simulink model "tanks_dis"  (R2021b)
settings: Solver=VariableStepAuto  StartTime=0.0  StopTime=200  RelTol=1e-3
values from neighbouring files (symbols this model uses):
  F = tf([K_pid*(Ti+Td*Ti*N), K_pid*(Ti*N +1),K_pid*N],[Ti, Ti*N 0])    [control_design.m]
  Ts = 4    [control_design.m]
  uss = alpha2/beta*sqrt(2*g*tank_init_h2)*100/15    [control_design.m]
  yss = 40    [control_design.m]
undefined symbols (not defined in the file or in its folder): A_discretized, B_discretized, C_discretized, D_discretized, tank_A1, tank_a1, tank_A2, tank_a2, tank_H1, tank_H2, tank_init_h1, tank_init_h2, tank_Kpump
settings Model: LastModifiedBy=rivaa
settings OptimizationCC: BlockReduction=off  BooleanDataType=off
settings DebuggingCC: SaveWithParameterizedLinksMsg=none  UnderspecifiedInitializationDetection=Classic  MergeDetectMultiDrivingBlocksExec=none  SignalResolutionControl=TryResolveAllWithWarning
settings HardwareCC: TargetUnknown=on
settings ModelReferenceCC: PropagateSignalLabelsOutOfModel=off

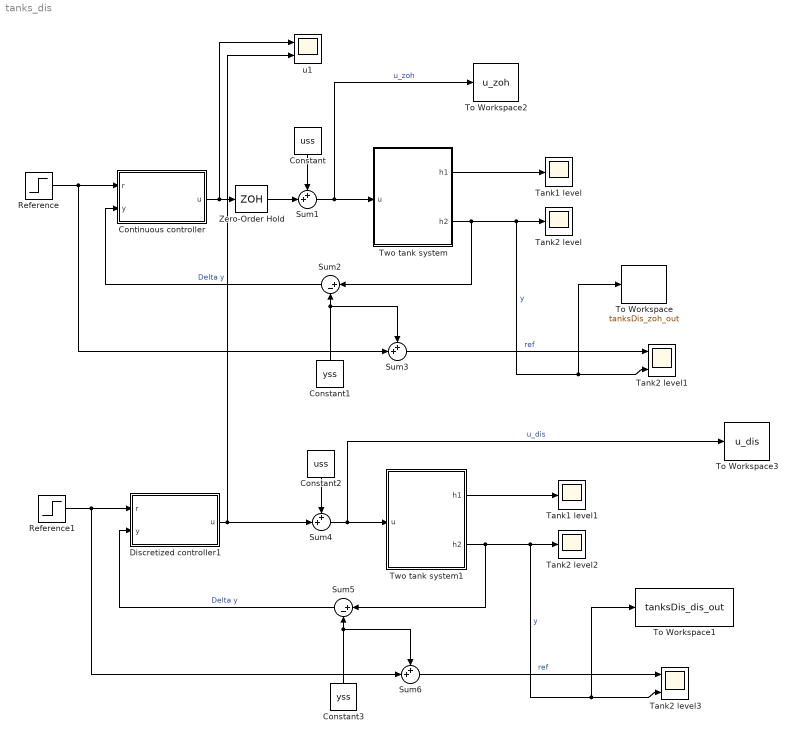
== system tanks_dis ==
  Constant : Constant  Value=uss
  Constant1 : Constant  Value=yss
  Constant2 : Constant  Value=uss
  Constant3 : Constant  Value=yss
  Continuous controller : Subsystem
  Discretized controller1 : Subsystem
  Reference : Step  Time=25  After=10  SampleTime=0
  Reference1 : Step  Time=25  After=10  SampleTime=0
  Sum{1,3..4,6} (4 alike) : Sum  Inputs=++|
  Sum2 : Sum  Inputs=|+-
  Sum5 : Sum  Inputs=|+-
  Tank1 level : Scope
  Tank1 level1 : Scope
  Tank2 level : Scope
  Tank2 level1 : Scope  NumInputPorts=2
  Tank2 level2 : Scope
  Tank2 level3 : Scope  NumInputPorts=2
  To Workspace : ToWorkspace  VariableName=tanksDis_zoh_out  SaveFormat=Structure With Time  SampleTime=-1
      settings: Save2DSignal=2-D array (concatenate along first dimension)
  To Workspace1 : ToWorkspace  VariableName=tanksDis_dis_out  SaveFormat=Structure With Time  SampleTime=-1
      settings: Save2DSignal=2-D array (concatenate along first dimension)
  To Workspace2 : ToWorkspace  VariableName=u_zoh  SaveFormat=Structure With Time  SampleTime=-1
      settings: Save2DSignal=2-D array (concatenate along first dimension)
  To Workspace3 : ToWorkspace  VariableName=u_dis  SaveFormat=Structure With Time  SampleTime=-1
      settings: Save2DSignal=2-D array (concatenate along first dimension)
  Two tank system : Subsystem
  Two tank system1 : Subsystem
  Zero-Order Hold : ZeroOrderHold  SampleTime=Ts
  u1 : Scope  NumInputPorts=2
  wires:
  Constant1/1 -> Sum3/1, Sum2/2
  Continuous controller/1(u) -> u1/1, Zero-Order Hold/1
  Constant/1 -> Sum1/1
  Two tank system/1(h1) -> Tank1 level/1
  Sum1/1 -> To Workspace2/1, Two tank system/1(u)  "u_zoh"
  Two tank system/2(h2) -> Sum2/1, To Workspace/1, Tank2 level1/2, Tank2 level/1  "y"
  Zero-Order Hold/1 -> Sum1/2
  Reference/1 -> Continuous controller/1(r), Sum3/2
  Sum3/1 -> Tank2 level1/1  "ref"
  Sum2/1 -> Continuous controller/2(y)  "Delta y"
  Sum5/1 -> Discretized controller1/2(y)  "Delta y"
  Sum6/1 -> Tank2 level3/1  "ref"
  Reference1/1 -> Discretized controller1/1(r), Sum6/2
  Discretized controller1/1(u) -> u1/2, Sum4/2
  Two tank system1/2(h2) -> Tank2 level2/1, Tank2 level3/2, To Workspace1/1, Sum5/1  "y"
  Sum4/1 -> To Workspace3/1, Two tank system1/1(u)  "u_dis"
  Two tank system1/1(h1) -> Tank1 level1/1
  Constant2/1 -> Sum4/1
  Constant3/1 -> Sum5/2, Sum6/1

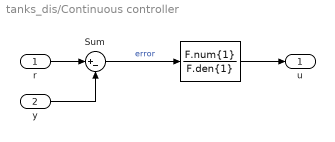
== system tanks_dis/Continuous controller ==
  r : Inport
  y : Inport  Port=2
  " " : TransferFcn  Numerator=F.num{1}  Denominator=F.den{1}
  Sum : Sum  Inputs=|+-  SaturateOnIntegerOverflow=on
  u : Outport
  wires:
  Sum/1 -> " "/1  "error"
  y/1 -> Sum/2
  r/1 -> Sum/1
  " "/1 -> u/1

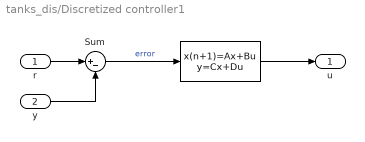
== system tanks_dis/Discretized controller1 ==
  r : Inport
  y : Inport  Port=2
  " " : DiscreteStateSpace  A=A_discretized  B=B_discretized  C=C_discretized  D=D_discretized  SampleTime=Ts
  Sum : Sum  Inputs=|+-  SaturateOnIntegerOverflow=on
  u : Outport
  wires:
  " "/1 -> u/1
  r/1 -> Sum/1
  y/1 -> Sum/2
  Sum/1 -> " "/1  "error"

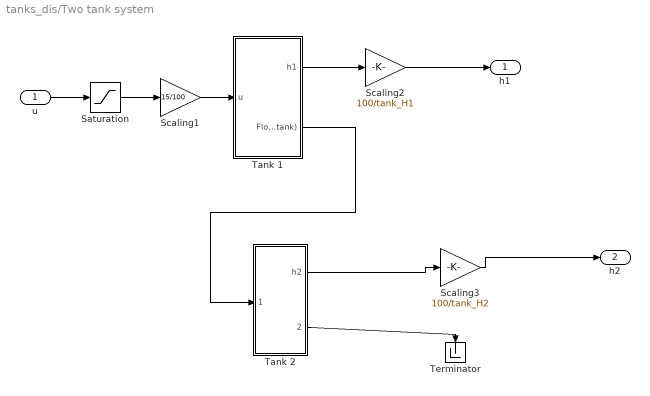
== system tanks_dis/Two tank system ==
  u : Inport
  Saturation : Saturate  UpperLimit=100  LowerLimit=-0
  Scaling1 : Gain  Gain=15/100  SaturateOnIntegerOverflow=on  OutDataTypeStr=Inherit: Same as input  ParamDataTypeStr=Inherit: Same as input
  Scaling2 : Gain  Gain=100/tank_H1  SaturateOnIntegerOverflow=on  OutDataTypeStr=Inherit: Same as input  ParamDataTypeStr=Inherit: Same as input
  Scaling3 : Gain  Gain=100/tank_H2  SaturateOnIntegerOverflow=on  OutDataTypeStr=Inherit: Same as input  ParamDataTypeStr=Inherit: Same as input
  Tank 1 : Subsystem
  Tank 2 : Subsystem
  Terminator : Terminator
  h1 : Outport
  h2 : Outport  Port=2
  wires:
  Tank 2/1(h2) -> Scaling3/1
  Tank 2/2(Flow out) -> Terminator/1
  u/1 -> Saturation/1
  Tank 1/1(h1) -> Scaling2/1
  Tank 1/2(Flow out  (to lower tank)) -> Tank 2/1(From upper tank)
  Scaling2/1 -> h1/1
  Scaling3/1 -> h2/1
  Scaling1/1 -> Tank 1/1(u)
  Saturation/1 -> Scaling1/1

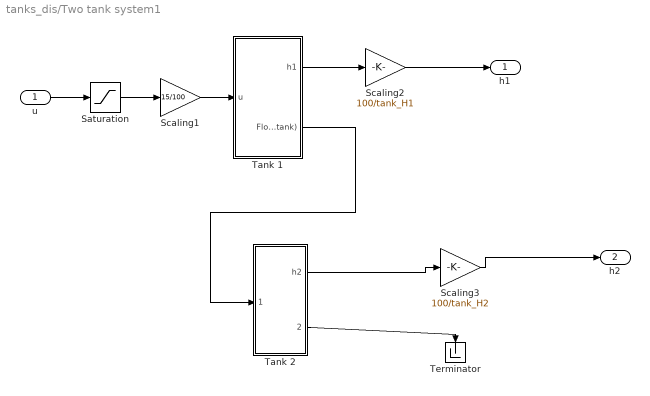
== system tanks_dis/Two tank system1 ==
  u : Inport
  Saturation : Saturate  UpperLimit=100  LowerLimit=-0
  Scaling1 : Gain  Gain=15/100  SaturateOnIntegerOverflow=on  OutDataTypeStr=Inherit: Same as input  ParamDataTypeStr=Inherit: Same as input
  Scaling2 : Gain  Gain=100/tank_H1  SaturateOnIntegerOverflow=on  OutDataTypeStr=Inherit: Same as input  ParamDataTypeStr=Inherit: Same as input
  Scaling3 : Gain  Gain=100/tank_H2  SaturateOnIntegerOverflow=on  OutDataTypeStr=Inherit: Same as input  ParamDataTypeStr=Inherit: Same as input
  Tank 1 : Subsystem
  Tank 2 : Subsystem
  Terminator : Terminator
  h1 : Outport
  h2 : Outport  Port=2
  wires:
  Saturation/1 -> Scaling1/1
  Scaling1/1 -> Tank 1/1(u)
  Scaling3/1 -> h2/1
  Scaling2/1 -> h1/1
  Tank 1/2(Flow out  (to lower tank)) -> Tank 2/1(From upper tank)
  Tank 1/1(h1) -> Scaling2/1
  u/1 -> Saturation/1
  Tank 2/2(Flow out) -> Terminator/1
  Tank 2/1(h2) -> Scaling3/1

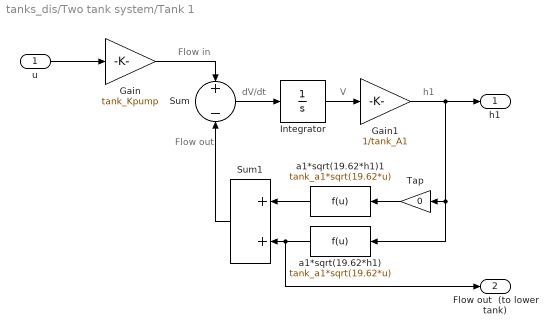
== system tanks_dis/Two tank system/Tank 1 ==
  note: h1
  note: V
  note: dV/dt
  note: Flow out
  note: Flow in
  u : Inport
  Gain : Gain  Gain=tank_Kpump  SaturateOnIntegerOverflow=on  OutDataTypeStr=Inherit: Same as input  ParamDataTypeStr=Inherit: Same as input
  Gain1 : Gain  Gain=1/tank_A1  SaturateOnIntegerOverflow=on  OutDataTypeStr=Inherit: Same as input  ParamDataTypeStr=Inherit: Same as input
  Integrator : Integrator  InitialCondition=tank_init_h1*tank_A1  LimitOutput=on  UpperSaturationLimit=tank_H1*tank_A1  LowerSaturationLimit=0
  Sum : Sum  Inputs=+-  InputSameDT=on  SaturateOnIntegerOverflow=on  OutDataTypeStr=Inherit: Same as first input
  Sum1 : Sum  InputSameDT=on  SaturateOnIntegerOverflow=on  OutDataTypeStr=Inherit: Same as first input
  Tap : Gain  Gain=0  SaturateOnIntegerOverflow=on  OutDataTypeStr=Inherit: Same as input  ParamDataTypeStr=Inherit: Same as input
  a1*sqrt(19.62*h1) : Fcn  Expr=tank_a1*sqrt(19.62*u)
  a1*sqrt(19.62*h1)1 : Fcn  Expr=tank_a1*sqrt(19.62*u)
  h1 : Outport
  Flow out  (to lower tank) : Outport  Port=2
  wires:
  Gain1/1 -> Tap/1, a1*sqrt(19.62*h1)/1, h1/1
  Integrator/1 -> Gain1/1
  Sum/1 -> Integrator/1
  Gain/1 -> Sum/1
  u/1 -> Gain/1
  a1*sqrt(19.62*h1)/1 -> Flow out  (to lower tank)/1, Sum1/2
  a1*sqrt(19.62*h1)1/1 -> Sum1/1
  Sum1/1 -> Sum/2
  Tap/1 -> a1*sqrt(19.62*h1)1/1

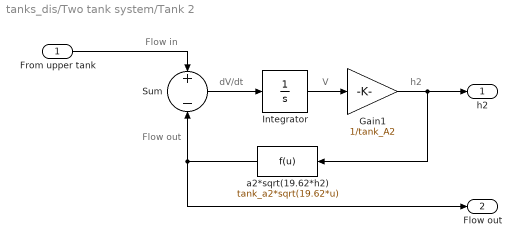
== system tanks_dis/Two tank system/Tank 2 ==
  note: Flow in
  note: Flow out
  note: dV/dt
  note: V
  note: h2
  From upper tank : Inport
  Gain1 : Gain  Gain=1/tank_A2  SaturateOnIntegerOverflow=on  OutDataTypeStr=Inherit: Same as input  ParamDataTypeStr=Inherit: Same as input
  Integrator : Integrator  InitialCondition=tank_init_h2*tank_A2  LimitOutput=on  UpperSaturationLimit=tank_H2*tank_A2  LowerSaturationLimit=0
  Sum : Sum  Inputs=+-  InputSameDT=on  SaturateOnIntegerOverflow=on  OutDataTypeStr=Inherit: Same as first input
  a2*sqrt(19.62*h2) : Fcn  Expr=tank_a2*sqrt(19.62*u)
  h2 : Outport
  Flow out : Outport  Port=2
  wires:
  Sum/1 -> Integrator/1
  Integrator/1 -> Gain1/1
  Gain1/1 -> h2/1, a2*sqrt(19.62*h2)/1
  a2*sqrt(19.62*h2)/1 -> Sum/2, Flow out/1
  From upper tank/1 -> Sum/1

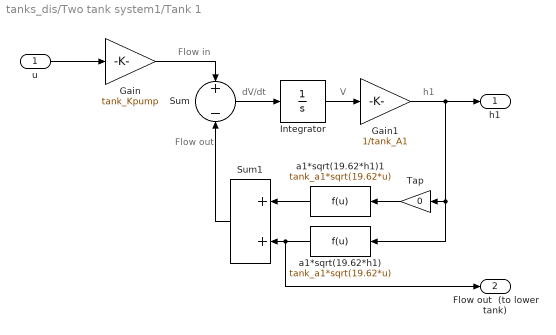
== system tanks_dis/Two tank system1/Tank 1 ==
  note: Flow in
  note: Flow out
  note: dV/dt
  note: V
  note: h1
  u : Inport
  Gain : Gain  Gain=tank_Kpump  SaturateOnIntegerOverflow=on  OutDataTypeStr=Inherit: Same as input  ParamDataTypeStr=Inherit: Same as input
  Gain1 : Gain  Gain=1/tank_A1  SaturateOnIntegerOverflow=on  OutDataTypeStr=Inherit: Same as input  ParamDataTypeStr=Inherit: Same as input
  Integrator : Integrator  InitialCondition=tank_init_h1*tank_A1  LimitOutput=on  UpperSaturationLimit=tank_H1*tank_A1  LowerSaturationLimit=0
  Sum : Sum  Inputs=+-  InputSameDT=on  SaturateOnIntegerOverflow=on  OutDataTypeStr=Inherit: Same as first input
  Sum1 : Sum  InputSameDT=on  SaturateOnIntegerOverflow=on  OutDataTypeStr=Inherit: Same as first input
  Tap : Gain  Gain=0  SaturateOnIntegerOverflow=on  OutDataTypeStr=Inherit: Same as input  ParamDataTypeStr=Inherit: Same as input
  a1*sqrt(19.62*h1) : Fcn  Expr=tank_a1*sqrt(19.62*u)
  a1*sqrt(19.62*h1)1 : Fcn  Expr=tank_a1*sqrt(19.62*u)
  h1 : Outport
  Flow out  (to lower tank) : Outport  Port=2
  wires:
  Tap/1 -> a1*sqrt(19.62*h1)1/1
  Sum1/1 -> Sum/2
  a1*sqrt(19.62*h1)1/1 -> Sum1/1
  a1*sqrt(19.62*h1)/1 -> Sum1/2, Flow out  (to lower tank)/1
  u/1 -> Gain/1
  Gain/1 -> Sum/1
  Sum/1 -> Integrator/1
  Integrator/1 -> Gain1/1
  Gain1/1 -> h1/1, a1*sqrt(19.62*h1)/1, Tap/1

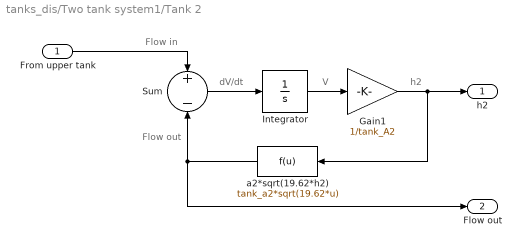
== system tanks_dis/Two tank system1/Tank 2 ==
  note: h2
  note: V
  note: dV/dt
  note: Flow out
  note: Flow in
  From upper tank : Inport
  Gain1 : Gain  Gain=1/tank_A2  SaturateOnIntegerOverflow=on  OutDataTypeStr=Inherit: Same as input  ParamDataTypeStr=Inherit: Same as input
  Integrator : Integrator  InitialCondition=tank_init_h2*tank_A2  LimitOutput=on  UpperSaturationLimit=tank_H2*tank_A2  LowerSaturationLimit=0
  Sum : Sum  Inputs=+-  InputSameDT=on  SaturateOnIntegerOverflow=on  OutDataTypeStr=Inherit: Same as first input
  a2*sqrt(19.62*h2) : Fcn  Expr=tank_a2*sqrt(19.62*u)
  h2 : Outport
  Flow out : Outport  Port=2
  wires:
  From upper tank/1 -> Sum/1
  a2*sqrt(19.62*h2)/1 -> Flow out/1, Sum/2
  Gain1/1 -> a2*sqrt(19.62*h2)/1, h2/1
  Integrator/1 -> Gain1/1
  Sum/1 -> Integrator/1
